simulink model "FOC_basic2_VoltageCtrl"  (R2020b)
settings: Solver=FixedStepAuto  StartTime=0.0  StopTime=inf  FixedStep=Ts  MaxStep=0.0005  RelTol=1e-3
InitFcn:
  | FOC_basic;
undefined symbols (not defined in the file): motor, Ts
libraries: mcbcontrolslib x2, autolibpmsminterior x1
settings Model: Creator=k  LastModifiedBy=k

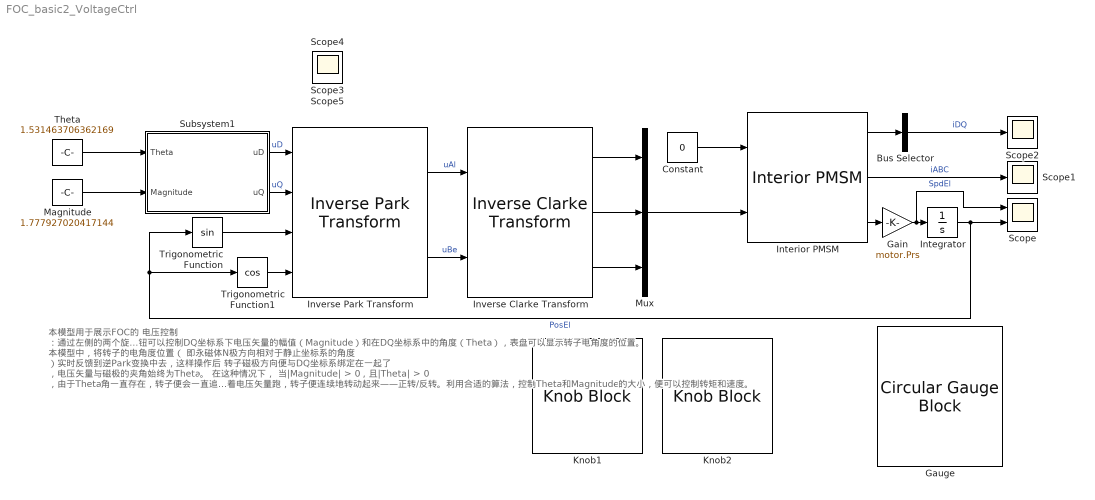
== system FOC_basic2_VoltageCtrl ==
  note: 本模型用于展示FOC的 电压控制 ：通过左侧的两个旋钮可以控制DQ坐标系下电压矢量的幅值（Magnitude）和在DQ坐标系中的角度（Theta），表盘可以显示转子电角度的位置。
      |
      | 本模型中，将转子的电角度位置（ 即永磁体N极方向相对于静止坐标系的角度 ）实时反馈到逆Park变换中去，这样操作后 转子磁极方向便与DQ坐标系绑定在一起了 ，电压矢量与磁极的夹角始终为Theta。
      |
      | 在这种情况下， 当|Magnitude| > 0，且|Theta| > 0 ，由于Theta角一直存在，转子便会一直追着电压矢量跑，转子便连续地转动起来——正转/反转。利用合适的算法，控制Theta和Magnitude的大小，便可以控制转矩和速度。
  Bus Selector : BusSelector  OutputSignals=IdSync,IqSync  OutputAsBus=on
  Constant : Constant  Value=0
  Gain : Gain  Gain=motor.Prs
  Gauge : CircularGaugeBlock  ScaleMin=-3.14  ScaleMax=3.14  TickInterval=1.57
  Integrator : Integrator  WrapState=on
  Interior PMSM : autolibpmsminterior/Interior PMSM  port_config=Torque  sim_type=Continuous  Ts=0.001  P=motor.Prs  Rs=motor.Rs  Ldq=[motor.Ld motor.Lq]  KConstText=Permanent flux linkage constant (lambda_pm):  lambda_pm=motor.Flux  Ke=159.9771  mechanical=[motor.J, motor.B, motor.Tf]  idq0=[0 0]  theta_init=0  omega_init=0  KConst=motor.Flux  lambda_pm_calc=motor.Flux  Kt=0.07  RefBlkName='autolibpmsminterior/Interior PMSM'  aMode=5
      settings: SourceProductBaseCode=PW,MT,UV,VE,VP
  Inverse Clarke Transform : mcbcontrolslib/Inverse Clarke Transform
      settings: SourceProductBaseCode=MT
  Inverse Park Transform : mcbcontrolslib/Inverse Park Transform  AxisAlignment=D-axis
  Knob1 : KnobBlock  ScaleMin=-12  ScaleMax=12
  Knob2 : KnobBlock  ScaleMin=-3.14  ScaleMax=3.14  TickInterval=1.57
  Magnitude : Constant  Value=1.777927020417144
  Mux : Mux  Inputs=3
  Scope : Scope  NumInputPorts=2
  Scope{1..5} (5 alike) : Scope
  Subsystem1 : Subsystem
      mask Display: disp('Theta & Magnitue \n to Vector');
  Theta : Constant  Value=1.531463706362169
  Trigonometric Function : Trigonometry
  Trigonometric Function1 : Trigonometry  Operator=cos
  wires:
  Trigonometric Function/1 -> Inverse Park Transform/3
  Trigonometric Function1/1 -> Inverse Park Transform/4
  Inverse Park Transform/1 -> Inverse Clarke Transform/1  "uAl"
  Inverse Park Transform/2 -> Inverse Clarke Transform/2  "uBe"
  Subsystem1/1(uD) -> Inverse Park Transform/1  "uD"
  Subsystem1/2(uQ) -> Inverse Park Transform/2  "uQ"
  Theta/1 -> Subsystem1/1(Theta)
  Magnitude/1 -> Subsystem1/2(Magnitude)
  Bus Selector/1 -> Scope2/1  "iDQ"
  Interior PMSM/3 -> Gain/1
  Interior PMSM/1 -> Bus Selector/1
  Interior PMSM/2 -> Scope1/1  "iABC"
  Inverse Clarke Transform/3 -> Mux/3
  Gain/1 -> Scope/1, Integrator/1  "SpdEl"
  Inverse Clarke Transform/1 -> Mux/1
  Constant/1 -> Interior PMSM/1
  Inverse Clarke Transform/2 -> Mux/2
  Integrator/1 -> Trigonometric Function/1, Trigonometric Function1/1, Scope/2  "PosEl"
  Mux/1 -> Interior PMSM/2

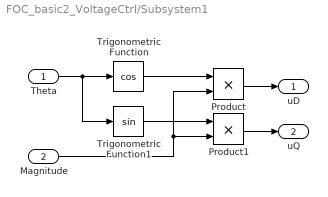
== system FOC_basic2_VoltageCtrl/Subsystem1 ==
  Theta : Inport  SampleTime=Ts
  Magnitude : Inport  Port=2  SampleTime=Ts
  Product : Product
  Product1 : Product
  Trigonometric Function : Trigonometry  Operator=cos
  Trigonometric Function1 : Trigonometry
  uD : Outport
  uQ : Outport  Port=2
  wires:
  Product/1 -> uD/1
  Product1/1 -> uQ/1
  Trigonometric Function/1 -> Product/1
  Trigonometric Function1/1 -> Product1/1
  Magnitude/1 -> Product/2, Product1/2
  Theta/1 -> Trigonometric Function1/1, Trigonometric Function/1
